simulink model "accurateTiltingModel2"  (R2022b)
settings: Solver=ode4  StartTime=0.0  StopTime=10.0  FixedStep=0.001  RelTol=1e-3
undefined symbols (not defined in the file): Angle, Axis, I_b, I_i, k_m
libraries: robotcorelib x8, matrix_library x5, slpidlib x2
settings Model: Creator=pozzan  LastModifiedBy=pozzan

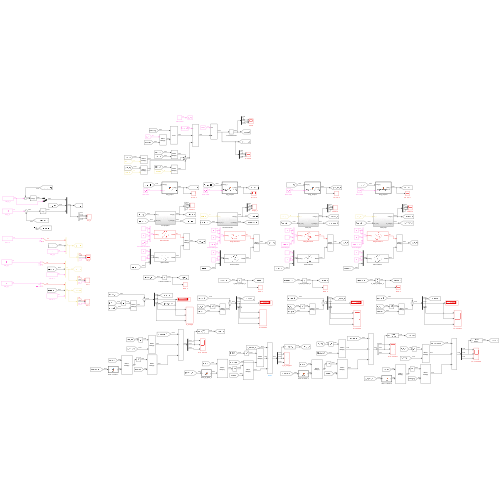
[thumbnail: Simulink's stored preview of the top-level diagram]
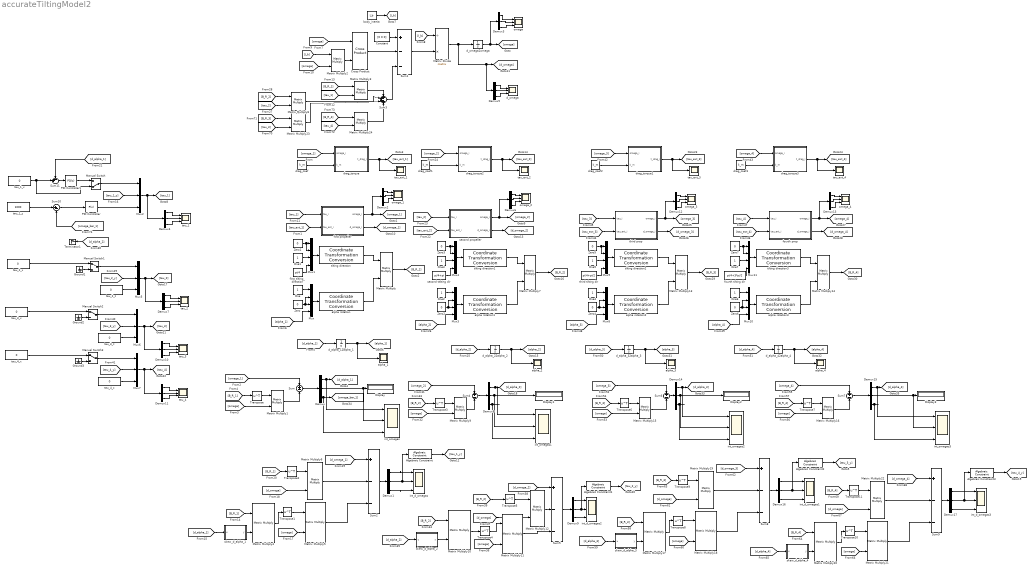
== system accurateTiltingModel2 ==
  Algebraic Constraint{,1..3} (4 alike) : AlgebraicConstraint
  Constant : Constant  Value=[0 0 0]
  Cross Product : matrix_library/Cross Product
  Demux{,1..17} (18 alike) : Demux  Outputs=3
  Display{,1..3} (4 alike) : Display
  Ground1 : Ground
  Ground2 : Ground
  Ground3 : Ground
  Manual Switch : ManualSwitch  CurrentSetting=0
  Manual Switch1 : ManualSwitch
  Manual Switch2 : ManualSwitch
  Manual Switch3 : ManualSwitch
  Matrix Divide : Product  Inputs=/*  Multiplication=Matrix(*)
  Matrix Multiply{,1..24} (25 alike) : Product  Multiplication=Matrix(*)
  Mux{,1,3..4,8..11} (8 alike) : Mux
  Mux{2,5..7} (4 alike) : Mux  Inputs=3
  One{,1..7} (8 alike) : Constant  OutDataTypeStr=Inherit: Inherit via back propagation
  PID Controller : slpidlib/PID Controller  Controller=P  Form=Parallel  TimeDomain=Continuous-time  UseExternalTs=off  SampleTime=-1  IntegratorMethod=Forward Euler  FilterMethod=Forward Euler  ControllerParametersSource=internal  P=0.01  I=1  UseKiTs=off  D=0  N=100  UseFilter=on  TunerSelectOption=Transfer Function Based (PID Tuner App)  InitialConditionSource=internal  InitialConditionForIntegrator=0  InitialConditionForFilter=0  DifferentiatorICPrevScaledInput=0  ExternalReset=none  TrackingMode=off  Kt=1  LimitOutput=off  SatLimitsSource=internal  UpperSaturationLimit=inf  LowerSaturationLimit=-inf  LinearizeAsGain=on  AntiWindupMode=none  Kb=1  LimitIntegrator=off  UpperIntegratorSaturationLimit=inf  LowerIntegratorSaturationLimit=-inf  POutMin=[]  POutMax=[]  IOutMin=[]  IOutMax=[]  DOutMin=[]  DOutMax=[]  NOutMin=[]  NOutMax=[]  SumOutMin=[]  SumOutMax=[]  SaturationOutMin=[]  SaturationOutMax=[]  PParamMin=[]  PParamMax=[]  IParamMin=[]  IParamMax=[]  DParamMin=[]  DParamMax=[]  NParamMin=[]  NParamMax=[]  KbParamMin=[]  KbParamMax=[]  KtParamMin=[]  KtParamMax=[]  KbOutMin=[]  KbOutMax=[]  KtOutMin=[]  KtOutMax=[]  IntegratorOutMin=[]  IntegratorOutMax=[]  FilterOutMin=[]  FilterOutMax=[]  SumI1OutMin=[]  SumI1OutMax=[]  SumI2OutMin=[]  SumI2OutMax=[]  SumI3OutMin=[]  SumI3OutMax=[]  SumI4OutMin=[]  SumI4OutMax=[]  SumDOutMin=[]  SumDOutMax=[]  DifferentiatorOutMin=[]  DifferentiatorOutMax=[]  FilterDiffOutCoefMin=[]  FilterDiffOutCoefMax=[]  ReciprocalOutMin=[]  ReciprocalOutMax=[]  SumDenOutMin=[]  SumDenOutMax=[]  SumNumOutMin=[]  SumNumOutMax=[]  DivideOutMin=[]  DivideOutMax=[]  UdiffTsProdOutMin=[]  UdiffTsProdOutMax=[]  NTsProdOutMin=[]  NTsProdOutMax=[]  UintegralTsProdOutMin=[]  UintegralTsProdOutMax=[]  UngainTsProdOutMin=[]  UngainTsProdOutMax=[]  ClampingZeroOutDataTypeStr=Inherit: Inherit via back propagation  ClampingZeroOutMin=[]  ClampingZeroOutMax=[]  FilterDenConstantOutDataTypeStr=Inherit: Inherit via back propagation  FilterDenConstantOutMin=[]  FilterDenConstantOutMax=[]  PCopyOutDataTypeStr=Inherit: Inherit via back propagation  PCopyOutMin=[]  PCopyOutMax=[]  NCopyOutDataTypeStr=Inherit: Inherit via back propagation  NCopyOutMin=[]  NCopyOutMax=[]  IntegratorContinuousStateAttributes=''  IntegratorStateMustResolveToSignalObject=off  IntegratorRTWStateStorageClass=Auto  FilterContinuousStateAttributes=''  FilterStateMustResolveToSignalObject=off  FilterRTWStateStorageClass=Auto  ParallelPVariant=InternalParameters  IdealPVariant=Disabled  IVariant=Disabled  DVariant=Disabled  IntegratorVariant=Disabled  SatVariant=Disabled  AWVariant=Disabled  PCopyVariant=Disabled  TRVariant=Disabled  FdbkBlocksVariant=Forward  IdealPFdbkVariant=Disabled  SatFdbkVariant=Disabled  DerivativeFilterVariant=Disabled  NVariant=Disabled  NCopyVariant=Disabled_SignalSpec  FilterICVariant=Disabled  IntegratorICVariant=Disabled  ExternalResetVariant=Disabled  TRSumVariant=Passthrough  SumFdbkVariant=Disabled  SumVariant=Passthrough_P  TsampFilterVariant=InternalTs  TsampNgainVariant=Passthrough  TsampIntegralVariant=Disabled_SignalSpec  ExternalSaturationOutDataTypeStr=Inherit: Same as second input
  PID Controller1 : slpidlib/PID Controller  Controller=PD  Form=Parallel  TimeDomain=Continuous-time  UseExternalTs=off  SampleTime=-1  IntegratorMethod=Forward Euler  FilterMethod=Forward Euler  ControllerParametersSource=internal  P=0.01  I=1  UseKiTs=off  D=0.01  N=100  UseFilter=on  TunerSelectOption=Transfer Function Based (PID Tuner App)  InitialConditionSource=internal  InitialConditionForIntegrator=0  InitialConditionForFilter=0  DifferentiatorICPrevScaledInput=0  ExternalReset=none  TrackingMode=off  Kt=1  LimitOutput=off  SatLimitsSource=internal  UpperSaturationLimit=inf  LowerSaturationLimit=-inf  LinearizeAsGain=on  AntiWindupMode=none  Kb=1  LimitIntegrator=off  UpperIntegratorSaturationLimit=inf  LowerIntegratorSaturationLimit=-inf  POutMin=[]  POutMax=[]  IOutMin=[]  IOutMax=[]  DOutMin=[]  DOutMax=[]  NOutMin=[]  NOutMax=[]  SumOutMin=[]  SumOutMax=[]  SaturationOutMin=[]  SaturationOutMax=[]  PParamMin=[]  PParamMax=[]  IParamMin=[]  IParamMax=[]  DParamMin=[]  DParamMax=[]  NParamMin=[]  NParamMax=[]  KbParamMin=[]  KbParamMax=[]  KtParamMin=[]  KtParamMax=[]  KbOutMin=[]  KbOutMax=[]  KtOutMin=[]  KtOutMax=[]  IntegratorOutMin=[]  IntegratorOutMax=[]  FilterOutMin=[]  FilterOutMax=[]  SumI1OutMin=[]  SumI1OutMax=[]  SumI2OutMin=[]  SumI2OutMax=[]  SumI3OutMin=[]  SumI3OutMax=[]  SumI4OutMin=[]  SumI4OutMax=[]  SumDOutMin=[]  SumDOutMax=[]  DifferentiatorOutMin=[]  DifferentiatorOutMax=[]  FilterDiffOutCoefMin=[]  FilterDiffOutCoefMax=[]  ReciprocalOutMin=[]  ReciprocalOutMax=[]  SumDenOutMin=[]  SumDenOutMax=[]  SumNumOutMin=[]  SumNumOutMax=[]  DivideOutMin=[]  DivideOutMax=[]  UdiffTsProdOutMin=[]  UdiffTsProdOutMax=[]  NTsProdOutMin=[]  NTsProdOutMax=[]  UintegralTsProdOutMin=[]  UintegralTsProdOutMax=[]  UngainTsProdOutMin=[]  UngainTsProdOutMax=[]  ClampingZeroOutDataTypeStr=Inherit: Inherit via back propagation  ClampingZeroOutMin=[]  ClampingZeroOutMax=[]  FilterDenConstantOutDataTypeStr=Inherit: Inherit via back propagation  FilterDenConstantOutMin=[]  FilterDenConstantOutMax=[]  PCopyOutDataTypeStr=Inherit: Inherit via back propagation  PCopyOutMin=[]  PCopyOutMax=[]  NCopyOutDataTypeStr=Inherit: Inherit via back propagation  NCopyOutMin=[]  NCopyOutMax=[]  IntegratorContinuousStateAttributes=''  IntegratorStateMustResolveToSignalObject=off  IntegratorRTWStateStorageClass=Auto  FilterContinuousStateAttributes=''  FilterStateMustResolveToSignalObject=off  FilterRTWStateStorageClass=Auto  ParallelPVariant=InternalParameters  IdealPVariant=Disabled  IVariant=Disabled  DVariant=InternalParameters  IntegratorVariant=Disabled  SatVariant=Disabled  AWVariant=Disabled  PCopyVariant=Disabled  TRVariant=Disabled  FdbkBlocksVariant=Forward  IdealPFdbkVariant=Disabled  SatFdbkVariant=Disabled  DerivativeFilterVariant=ContFilter  NVariant=InternalParameters  NCopyVariant=Disabled  FilterICVariant=InternalICsFilter  IntegratorICVariant=Disabled  ExternalResetVariant=Disabled  TRSumVariant=Passthrough  SumFdbkVariant=Disabled  SumVariant=Sum_PD  TsampFilterVariant=InternalTs  TsampNgainVariant=Passthrough  TsampIntegralVariant=Disabled_SignalSpec  ExternalSaturationOutDataTypeStr=Inherit: Same as second input
  Sum{,4,6..7} (4 alike) : Sum  Inputs=+-
  Sum{1..2,5,8..9} (5 alike) : Sum  Inputs=+--
  Sum10 : Sum  Inputs=|+-
  Sum11 : Sum  Inputs=-+|
  Sum3 : Sum  Inputs=++++
  Terminator1 : Terminator
  Transpose{,1..11} (12 alike) : Math  Operator=transpose
  Zero{,1..7} (8 alike) : Constant  Value=0  OutDataTypeStr=Inherit: Inherit via back propagation
  alpha rotation{,1..3} (4 alike) : robotcorelib/Coordinate Transformation Conversion  InputRepresentation=Axis-Angle  InputEulerSequence=ZYX  ShowTrVecInputPort=on  OutputRepresentation=Rotation Matrix  OutputEulerSequence=ZYX  ShowTrVecOutputPort=on  SimulateUsing=Code generation
  alpha_{1..4} (4 alike) : Scope
  body_inertia : Constant  Value=I_b
  d_alpha_12alpha_1 : Integrator  InitialCondition=0.1
  d_alpha_22alpha_2 : Integrator  InitialCondition=0.1
  d_alpha_32alpha_3 : Integrator  InitialCondition=0.1
  d_alpha_42alpha_4 : Integrator  InitialCondition=0.1
  d_omega : Scope  NumInputPorts=3
  d_omega2omega : Integrator  InitialCondition=[0 0 0]
  drag_coef{,1..3} (4 alike) : Constant  Value=k_m
  drag_torque : MATLAB Function  TreatAsAtomicUnit=on
  drag_torque1 : MATLAB Function  TreatAsAtomicUnit=on
  drag_torque2 : MATLAB Function  TreatAsAtomicUnit=on
  drag_torque3 : MATLAB Function  TreatAsAtomicUnit=on
  first propeller : Subsystem
  first_tilting_direction : Constant  Value=pi/4
  fourth prop : Subsystem
  fourth tilting dir : Constant  Value=pi/4+3*pi/2
  int_d_omegas{,1..3} (4 alike) : Scope  NumInputPorts=3
  int_omegas{,1..3} (4 alike) : Scope  NumInputPorts=3
  omega : Scope  NumInputPorts=3
  omega_{1..4} (4 alike) : Scope  NumInputPorts=3
  second propeller : Subsystem
  second titlting dir : Constant  Value=pi/4+pi
  skew_d_alpha_1 : MATLAB Function  TreatAsAtomicUnit=on
  skew_d_alpha_2 : MATLAB Function  TreatAsAtomicUnit=on
  skew_d_alpha_3 : MATLAB Function  TreatAsAtomicUnit=on
  skew_d_alpha_4 : MATLAB Function  TreatAsAtomicUnit=on
  tau_{1..4} (4 alike) : Scope  NumInputPorts=3
  tau_1_x : Constant  Value=0
  tau_1_z : Constant  Value=1000
  tau_2_x : Constant  Value=0
  tau_2_z : Constant  Value=0
  tau_3_x : Constant  Value=0
  tau_3_z : Constant  Value=0
  tau_4_x : Constant  Value=0
  tau_4_z : Constant  Value=0
  tau_ext_{1..4} (4 alike) : Scope
  third prop : Subsystem
  third tilting dir : Constant  Value=pi/4+pi/2
  tilting direction{,1..3} (4 alike) : robotcorelib/Coordinate Transformation Conversion  InputRepresentation=Axis-Angle  InputEulerSequence=ZYX  ShowTrVecInputPort=on  OutputRepresentation=Rotation Matrix  OutputEulerSequence=ZYX  ShowTrVecOutputPort=on  SimulateUsing=Code generation
  wires:
  [omega_1] -> drag_torque/1(omega_i)
  Matrix Multiply/1 -> [B_R_1]
  Sum1/1 -> Matrix Divide/2
  tilting direction/1 -> Matrix Multiply/1
  first_tilting_direction/1 -> Mux1/4
  [omega] -> Cross Product/1
  Mux2/1 -> Demux4/1, [tau_1]
  Matrix Multiply1/1 -> Sum/2
  Matrix Multiply3/1 -> Sum3/1
  alpha rotation/1 -> Matrix Multiply/2
  Matrix Divide/1 -> Demux5/1, [d_omega], d_omega2omega/1
  Constant/1 -> Sum1/1
  [I_b] -> Matrix Multiply2/1
  Sum/1 -> Demux/1
  [omega] -> Matrix Multiply2/2
  Cross Product/1 -> Sum1/2
  drag_coef/1 -> drag_torque/2(k_m)
  Transpose/1 -> Matrix Multiply1/1
  [alpha_1] -> Mux/4
  One1/1 -> Mux1/3
  d_omega2omega/1 -> Demux3/1, [omega]
  Matrix Multiply2/1 -> Cross Product/2
  Demux/1 -> int_omegas/1, [d_alpha_1]
  drag_torque/1(t_drag_i) -> tau_ext_1/1, [tau_ext_1]
  body_inertia/1 -> [I_b]
  [d_alpha_1] -> d_alpha_12alpha_1/1
  Mux/1 -> alpha rotation/1
  [tau_ext_1] -> first propeller/2(tau_ext_i)
  [omega] -> Matrix Multiply1/2
  [omega_1] -> Sum/1
  d_alpha_12alpha_1/1 -> alpha_1/1, [alpha_1]
  Zero/1 -> Mux/2, Mux/3
  One/1 -> Mux/1
  Demux/3 -> [omega_bar_1], int_omegas/3
  first propeller/1(omega_i) -> Demux2/1, [omega_1]
  tau_1_z/1 -> Sum10/1
  Demux/2 -> int_omegas/2, Display/1
  Mux1/1 -> tilting direction/1
  [tau_1] -> Matrix Multiply3/2
  [tau_1] -> first propeller/1(tau_i)
  [B_R_1] -> Transpose/1
  Zero1/1 -> Mux1/1, Mux1/2
  [I_b] -> Matrix Divide/1
  [B_R_1] -> Matrix Multiply4/1
  [B_R_1] -> Matrix Multiply3/1
  [tau_1_y] -> Mux2/2
  first propeller/2(d_omega_i) -> [d_omega_1]
  [d_alpha_1] -> skew_d_alpha_1/1(u)
  skew_d_alpha_1/1(y) -> Matrix Multiply4/2
  [omega] -> Matrix Multiply5/2
  [d_omega_1] -> Sum2/1
  Transpose1/1 -> Matrix Multiply5/1
  Matrix Multiply4/1 -> Transpose1/1
  [B_R_1] -> Transpose2/1
  Transpose2/1 -> Matrix Multiply6/1
  [d_omega] -> Matrix Multiply6/2
  Matrix Multiply6/1 -> Sum2/2
  Sum2/1 -> Demux1/1
  Demux1/2 -> int_d_omegas/2, Algebraic Constraint/1
  Demux1/1 -> int_d_omegas/1
  Demux1/3 -> int_d_omegas/3
  Demux2/1 -> omega_1/1
  Demux2/2 -> omega_1/2
  Demux2/3 -> omega_1/3
  Demux3/3 -> omega/3
  Demux3/2 -> omega/2
  Demux3/1 -> omega/1
  Algebraic Constraint/1 -> [tau_1_y]
  Demux4/1 -> tau_1/1
  Demux4/2 -> tau_1/2
  Demux4/3 -> tau_1/3
  Matrix Multiply5/1 -> Sum2/3
  Demux5/1 -> d_omega/1
  Demux5/2 -> d_omega/2
  Demux5/3 -> d_omega/3
  Manual Switch/1 -> Mux2/1
  tau_1_x/1 -> Manual Switch/2, Sum11/2
  [d_alpha_1] -> Sum11/1
  Demux6/3 -> omega_2/3
  Demux6/2 -> omega_2/2
  Demux6/1 -> omega_2/1
  second propeller/2(d_omega_i) -> [d_omega_2]
  [tau_2] -> second propeller/1(tau_i)
  second propeller/1(omega_i) -> [omega_2], Demux6/1
  [tau_ext_2] -> second propeller/2(tau_ext_i)
  drag_torque2/1(t_drag_i) -> [tau_ext_2], tau_ext_2/1
  drag_coef1/1 -> drag_torque2/2(k_m)
  [omega_2] -> drag_torque2/1(omega_i)
  d_alpha_22alpha_2/1 -> [alpha_2], alpha_2/1
  [d_alpha_2] -> d_alpha_22alpha_2/1
  Zero3/1 -> Mux4/2, Mux4/1
  Mux4/1 -> tilting direction1/1
  One2/1 -> Mux3/1
  Zero2/1 -> Mux3/3, Mux3/2
  Mux3/1 -> alpha rotation1/1
  One3/1 -> Mux4/3
  [alpha_2] -> Mux3/4
  alpha rotation1/1 -> Matrix Multiply7/2
  second titlting dir/1 -> Mux4/4
  tilting direction1/1 -> Matrix Multiply7/1
  Matrix Multiply7/1 -> [B_R_2]
  Sum3/1 -> Sum1/3
  [B_R_2] -> Matrix Multiply8/1
  [tau_2] -> Matrix Multiply8/2
  Matrix Multiply8/1 -> Sum3/2
  [d_alpha_2] -> Terminator1/1
  Ground1/1 -> Manual Switch1/2
  tau_2_x/1 -> Manual Switch1/1
  Manual Switch1/1 -> Mux5/1
  Demux7/3 -> tau_2/3
  Demux7/2 -> tau_2/2
  Demux7/1 -> tau_2/1
  [tau_2_y] -> Mux5/2
  tau_2_z/1 -> Mux5/3
  Mux5/1 -> [tau_2], Demux7/1
  [B_R_2] -> Transpose3/1
  Demux8/2 -> Display1/1, int_omegas1/2
  Demux8/3 -> int_omegas1/3
  [omega_2] -> Sum4/1
  [omega] -> Matrix Multiply9/2
  Demux8/1 -> [d_alpha_2], int_omegas1/1
  Transpose3/1 -> Matrix Multiply9/1
  Sum4/1 -> Demux8/1
  Matrix Multiply9/1 -> Sum4/2
  Matrix Multiply11/1 -> Sum5/3
  Algebraic Constraint1/1 -> [tau_2_y]
  Demux9/3 -> int_d_omegas2/3
  Demux9/1 -> int_d_omegas2/1
  Demux9/2 -> int_d_omegas2/2, Algebraic Constraint1/1
  Sum5/1 -> Demux9/1
  Matrix Multiply12/1 -> Sum5/2
  [d_omega] -> Matrix Multiply12/2
  Transpose5/1 -> Matrix Multiply12/1
  [B_R_2] -> Transpose5/1
  Matrix Multiply10/1 -> Transpose4/1
  Transpose4/1 -> Matrix Multiply11/1
  [d_omega_2] -> Sum5/1
  [omega] -> Matrix Multiply11/2
  skew_d_alpha_2/1(y) -> Matrix Multiply10/2
  [d_alpha_2] -> skew_d_alpha_2/1(u)
  [B_R_2] -> Matrix Multiply10/1
  Mux6/1 -> Demux10/1, [tau_3]
  tau_3_z/1 -> Mux6/3
  [tau_3_y] -> Mux6/2
  Demux10/1 -> tau_3/1
  Demux10/2 -> tau_3/2
  Demux10/3 -> tau_3/3
  Manual Switch2/1 -> Mux6/1
  tau_3_x/1 -> Manual Switch2/1
  Ground2/1 -> Manual Switch2/2
  Ground3/1 -> Manual Switch3/2
  tau_4_x/1 -> Manual Switch3/1
  Manual Switch3/1 -> Mux7/1
  Demux11/3 -> tau_4/3
  Demux11/2 -> tau_4/2
  Demux11/1 -> tau_4/1
  [tau_4_y] -> Mux7/2
  tau_4_z/1 -> Mux7/3
  Mux7/1 -> [tau_4], Demux11/1
  drag_torque1/1(t_drag_i) -> [tau_ext_3], tau_ext_3/1
  drag_coef2/1 -> drag_torque1/2(k_m)
  [omega_3] -> drag_torque1/1(omega_i)
  [omega_4] -> drag_torque3/1(omega_i)
  drag_coef3/1 -> drag_torque3/2(k_m)
  drag_torque3/1(t_drag_i) -> tau_ext_4/1, [tau_ext_4]
  [tau_ext_3] -> third prop/2(tau_ext_i)
  Demux12/3 -> omega_3/3
  Demux12/2 -> omega_3/2
  third prop/1(omega_i) -> Demux12/1, [omega_3]
  Demux12/1 -> omega_3/1
  third prop/2(d_omega_i) -> [d_omega_3]
  [tau_3] -> third prop/1(tau_i)
  [tau_ext_4] -> fourth prop/2(tau_ext_i)
  Demux13/3 -> omega_4/3
  Demux13/2 -> omega_4/2
  fourth prop/1(omega_i) -> Demux13/1, [omega_4]
  Demux13/1 -> omega_4/1
  fourth prop/2(d_omega_i) -> [d_omega_4]
  [tau_4] -> fourth prop/1(tau_i)
  One4/1 -> Mux8/1
  One5/1 -> Mux9/3
  alpha rotation2/1 -> Matrix Multiply13/2
  Mux9/1 -> tilting direction2/1
  Zero4/1 -> Mux8/2, Mux8/3
  Mux8/1 -> alpha rotation2/1
  [alpha_3] -> Mux8/4
  third tilting dir/1 -> Mux9/4
  tilting direction2/1 -> Matrix Multiply13/1
  Matrix Multiply13/1 -> [B_R_3]
  Zero5/1 -> Mux9/1, Mux9/2
  One6/1 -> Mux10/1
  One7/1 -> Mux11/3
  alpha rotation3/1 -> Matrix Multiply14/2
  Mux11/1 -> tilting direction3/1
  Zero6/1 -> Mux10/2, Mux10/3
  Mux10/1 -> alpha rotation3/1
  [alpha_4] -> Mux10/4
  fourth tilting dir/1 -> Mux11/4
  tilting direction3/1 -> Matrix Multiply14/1
  Matrix Multiply14/1 -> [B_R_4]
  Zero7/1 -> Mux11/1, Mux11/2
  [d_alpha_3] -> d_alpha_32alpha_3/1
  d_alpha_32alpha_3/1 -> alpha_3/1, [alpha_3]
  [d_alpha_4] -> d_alpha_42alpha_4/1
  d_alpha_42alpha_4/1 -> alpha_4/1, [alpha_4]
  Demux14/3 -> int_omegas2/3
  Demux14/2 -> Display2/1, int_omegas2/2
  [omega_3] -> Sum6/1
  [omega] -> Matrix Multiply15/2
  Demux14/1 -> int_omegas2/1, [d_alpha_3]
  Transpose6/1 -> Matrix Multiply15/1
  Sum6/1 -> Demux14/1
  Matrix Multiply15/1 -> Sum6/2
  [B_R_3] -> Transpose6/1
  Demux15/3 -> int_omegas3/3
  Demux15/2 -> int_omegas3/2, Display3/1
  [omega_4] -> Sum7/1
  [omega] -> Matrix Multiply16/2
  Demux15/1 -> int_omegas3/1, [d_alpha_4]
  Transpose7/1 -> Matrix Multiply16/1
  Sum7/1 -> Demux15/1
  Matrix Multiply16/1 -> Sum7/2
  [B_R_4] -> Transpose7/1
  Matrix Multiply18/1 -> Sum8/3
  Algebraic Constraint2/1 -> [tau_3_y]
  Demux16/3 -> int_d_omegas1/3
  Demux16/1 -> int_d_omegas1/1
  Demux16/2 -> Algebraic Constraint2/1, int_d_omegas1/2
  Sum8/1 -> Demux16/1
  Matrix Multiply19/1 -> Sum8/2
  [d_omega] -> Matrix Multiply19/2
  Transpose9/1 -> Matrix Multiply19/1
  [B_R_3] -> Transpose9/1
  Matrix Multiply17/1 -> Transpose8/1
  Transpose8/1 -> Matrix Multiply18/1
  [d_omega_3] -> Sum8/1
  [omega] -> Matrix Multiply18/2
  skew_d_alpha_3/1(y) -> Matrix Multiply17/2
  [d_alpha_3] -> skew_d_alpha_3/1(u)
  [B_R_3] -> Matrix Multiply17/1
  [B_R_4] -> Matrix Multiply20/1
  [d_alpha_4] -> skew_d_alpha_4/1(u)
  skew_d_alpha_4/1(y) -> Matrix Multiply20/2
  [omega] -> Matrix Multiply21/2
  [d_omega_4] -> Sum9/1
  Transpose10/1 -> Matrix Multiply21/1
  Matrix Multiply20/1 -> Transpose10/1
  [B_R_4] -> Transpose11/1
  Transpose11/1 -> Matrix Multiply22/1
  [d_omega] -> Matrix Multiply22/2
  Matrix Multiply22/1 -> Sum9/2
  Sum9/1 -> Demux17/1
  Demux17/2 -> int_d_omegas3/2, Algebraic Constraint3/1
  Demux17/1 -> int_d_omegas3/1
  Demux17/3 -> int_d_omegas3/3
  Algebraic Constraint3/1 -> [tau_4_y]
  Matrix Multiply21/1 -> Sum9/3
  [tau_3] -> Matrix Multiply23/2
  [B_R_3] -> Matrix Multiply23/1
  Matrix Multiply23/1 -> Sum3/3
  [tau_4] -> Matrix Multiply24/2
  [B_R_4] -> Matrix Multiply24/1
  Matrix Multiply24/1 -> Sum3/4
  PID Controller/1 -> Mux2/3
  Sum10/1 -> PID Controller/1
  [omega_bar_1] -> Sum10/2
  Sum11/1 -> PID Controller1/1
  PID Controller1/1 -> Manual Switch/1

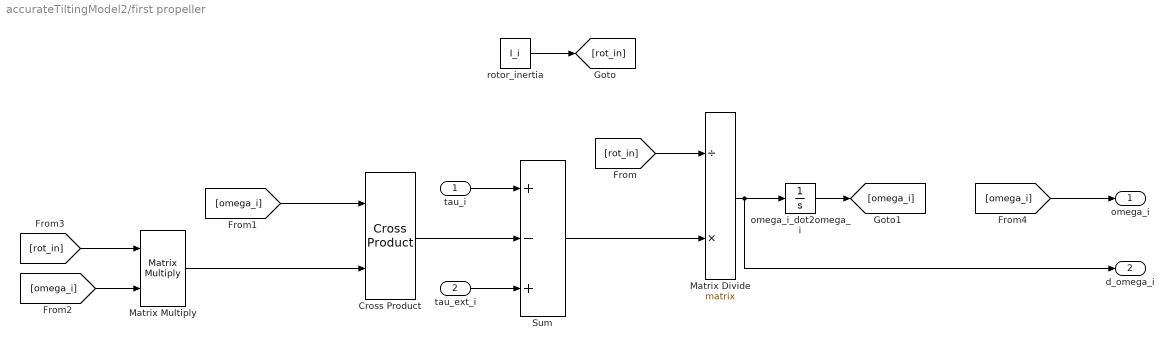
== system accurateTiltingModel2/first propeller ==
  tau_i : Inport  PortDimensions=3
  tau_ext_i : Inport  Port=2  PortDimensions=3
  Cross Product : matrix_library/Cross Product
  Matrix Divide : Product  Inputs=/*  Multiplication=Matrix(*)
  Matrix Multiply : Product  Multiplication=Matrix(*)
  Sum : Sum  Inputs=+-+
  omega_i_dot2omega_i : Integrator  InitialCondition=[0 0 0]
  rotor_inertia : Constant  Value=I_i
  omega_i : Outport
  d_omega_i : Outport  Port=2
  wires:
  [rot_in] -> Matrix Divide/1
  Matrix Divide/1 -> omega_i_dot2omega_i/1, d_omega_i/1
  omega_i_dot2omega_i/1 -> [omega_i]
  rotor_inertia/1 -> [rot_in]
  [omega_i] -> omega_i/1
  tau_ext_i/1 -> Sum/3
  [omega_i] -> Cross Product/1
  Cross Product/1 -> Sum/2
  Matrix Multiply/1 -> Cross Product/2
  [rot_in] -> Matrix Multiply/1
  [omega_i] -> Matrix Multiply/2
  Sum/1 -> Matrix Divide/2
  tau_i/1 -> Sum/1

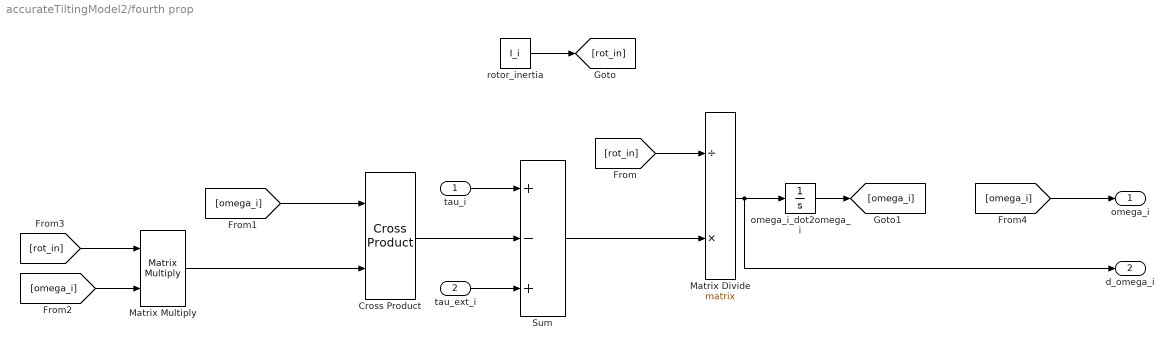
== system accurateTiltingModel2/fourth prop ==
  tau_i : Inport  PortDimensions=3
  tau_ext_i : Inport  Port=2  PortDimensions=3
  Cross Product : matrix_library/Cross Product
  Matrix Divide : Product  Inputs=/*  Multiplication=Matrix(*)
  Matrix Multiply : Product  Multiplication=Matrix(*)
  Sum : Sum  Inputs=+-+
  omega_i_dot2omega_i : Integrator  InitialCondition=[0 0 0]
  rotor_inertia : Constant  Value=I_i
  omega_i : Outport
  d_omega_i : Outport  Port=2
  wires:
  [rot_in] -> Matrix Divide/1
  Matrix Divide/1 -> omega_i_dot2omega_i/1, d_omega_i/1
  omega_i_dot2omega_i/1 -> [omega_i]
  rotor_inertia/1 -> [rot_in]
  [omega_i] -> omega_i/1
  tau_ext_i/1 -> Sum/3
  [omega_i] -> Cross Product/1
  Cross Product/1 -> Sum/2
  Matrix Multiply/1 -> Cross Product/2
  [rot_in] -> Matrix Multiply/1
  [omega_i] -> Matrix Multiply/2
  Sum/1 -> Matrix Divide/2
  tau_i/1 -> Sum/1

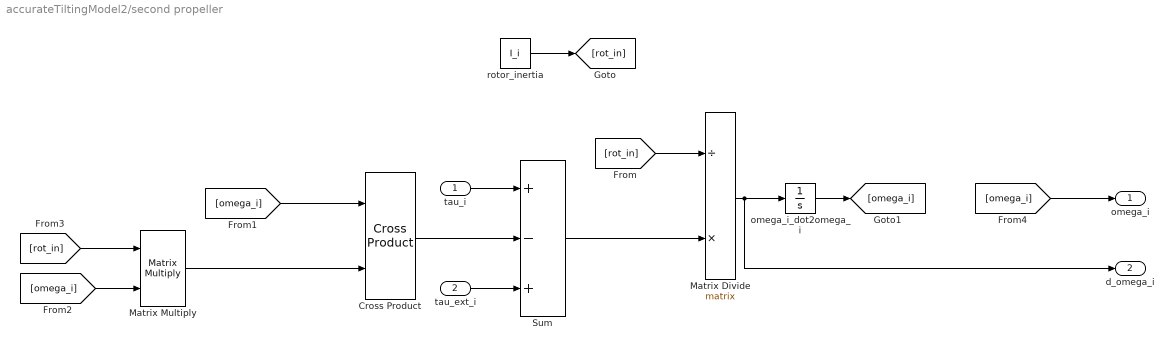
== system accurateTiltingModel2/second propeller ==
  tau_i : Inport  PortDimensions=3
  tau_ext_i : Inport  Port=2  PortDimensions=3
  Cross Product : matrix_library/Cross Product
  Matrix Divide : Product  Inputs=/*  Multiplication=Matrix(*)
  Matrix Multiply : Product  Multiplication=Matrix(*)
  Sum : Sum  Inputs=+-+
  omega_i_dot2omega_i : Integrator  InitialCondition=[0 0 0]
  rotor_inertia : Constant  Value=I_i
  omega_i : Outport
  d_omega_i : Outport  Port=2
  wires:
  tau_i/1 -> Sum/1
  Sum/1 -> Matrix Divide/2
  [omega_i] -> Matrix Multiply/2
  [rot_in] -> Matrix Multiply/1
  Matrix Multiply/1 -> Cross Product/2
  Cross Product/1 -> Sum/2
  [omega_i] -> Cross Product/1
  tau_ext_i/1 -> Sum/3
  [omega_i] -> omega_i/1
  rotor_inertia/1 -> [rot_in]
  omega_i_dot2omega_i/1 -> [omega_i]
  Matrix Divide/1 -> d_omega_i/1, omega_i_dot2omega_i/1
  [rot_in] -> Matrix Divide/1

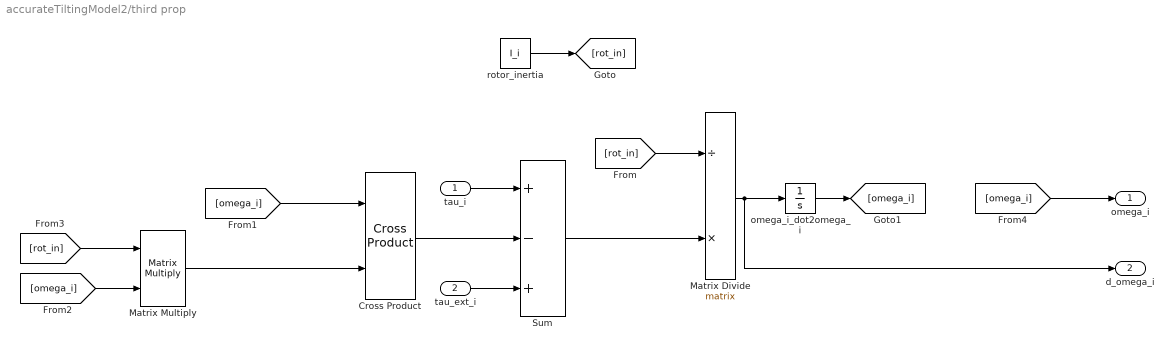
== system accurateTiltingModel2/third prop ==
  tau_i : Inport  PortDimensions=3
  tau_ext_i : Inport  Port=2  PortDimensions=3
  Cross Product : matrix_library/Cross Product
  Matrix Divide : Product  Inputs=/*  Multiplication=Matrix(*)
  Matrix Multiply : Product  Multiplication=Matrix(*)
  Sum : Sum  Inputs=+-+
  omega_i_dot2omega_i : Integrator  InitialCondition=[0 0 0]
  rotor_inertia : Constant  Value=I_i
  omega_i : Outport
  d_omega_i : Outport  Port=2
  wires:
  [rot_in] -> Matrix Divide/1
  Matrix Divide/1 -> omega_i_dot2omega_i/1, d_omega_i/1
  omega_i_dot2omega_i/1 -> [omega_i]
  rotor_inertia/1 -> [rot_in]
  [omega_i] -> omega_i/1
  tau_ext_i/1 -> Sum/3
  [omega_i] -> Cross Product/1
  Cross Product/1 -> Sum/2
  Matrix Multiply/1 -> Cross Product/2
  [rot_in] -> Matrix Multiply/1
  [omega_i] -> Matrix Multiply/2
  Sum/1 -> Matrix Divide/2
  tau_i/1 -> Sum/1

== matlab function accurateTiltingModel2/drag_torque ==
  data: omega_i input; k_m input; t_drag_i output
function t_drag_i = drag_from_spinning(omega_i, k_m)

t_drag_i = [0; 0; -k_m*omega_i(3)*abs(omega_i(3))];

== matlab function accurateTiltingModel2/drag_torque2 ==
  data: omega_i input; k_m input; t_drag_i output
function t_drag_i = drag_from_spinning(omega_i, k_m)

t_drag_i = [0; 0; -k_m*omega_i(3)*abs(omega_i(3))];

== matlab function accurateTiltingModel2/skew_d_alpha_2 ==
  data: u input; y output
function y = fcn(u)

y = [0 0 0
    0 0 -u
    0 u 0];

== matlab function accurateTiltingModel2/drag_torque1 ==
  data: omega_i input; k_m input; t_drag_i output
function t_drag_i = drag_from_spinning(omega_i, k_m)

t_drag_i = [0; 0; -k_m*omega_i(3)*abs(omega_i(3))];

== matlab function accurateTiltingModel2/drag_torque3 ==
  data: omega_i input; k_m input; t_drag_i output
function t_drag_i = drag_from_spinning(omega_i, k_m)

t_drag_i = [0; 0; -k_m*omega_i(3)*abs(omega_i(3))];

== matlab function accurateTiltingModel2/skew_d_alpha_3 ==
  data: u input; y output
function y = fcn(u)

y = [0 0 0
    0 0 -u
    0 u 0];

== matlab function accurateTiltingModel2/skew_d_alpha_4 ==
  data: u input; y output
function y = fcn(u)

y = [0 0 0
    0 0 -u
    0 u 0];

== matlab function accurateTiltingModel2/skew_d_alpha_1 ==
  data: u input; y output
function y = fcn(u)

y = [0 0 0
    0 0 -u
    0 u 0];
